simulink model "SatelliteDynamicsAndKinematics_Model"  (R2024a)
settings: Solver=VariableStepAuto  StartTime=0.0  StopTime=10.0  RelTol=1e-3
values from neighbouring files (symbols this model uses):
  sat = satellite_params()    [init_SAR_AOCS.m]
undefined symbols (not defined in the file or in its folder): initial
libraries: sharedtransform x3, matrix_library x1, aerolibutil x1, simulink_extras x1
settings Model: Creator=hendr  LastModifiedBy=hendr

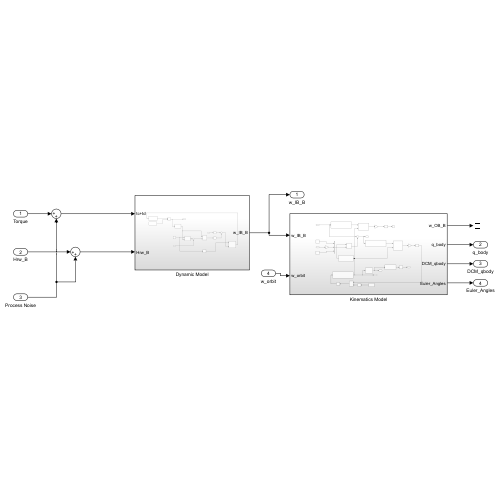
[thumbnail: Simulink's stored preview of the top-level diagram]
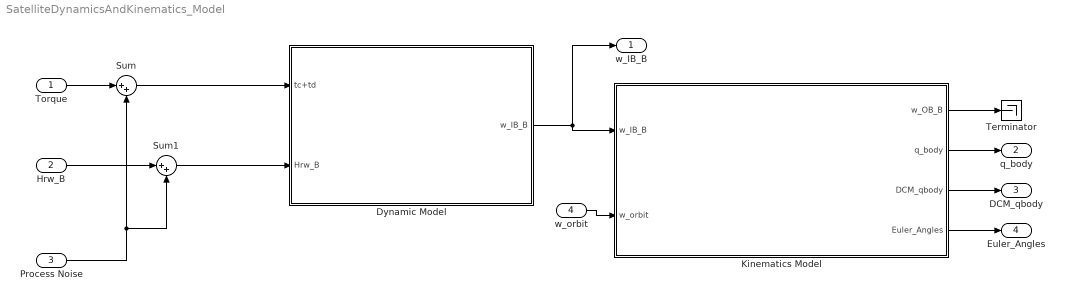
== system SatelliteDynamicsAndKinematics_Model ==
  Torque : Inport
  Hrw_B : Inport  Port=2
  Process Noise : Inport  Port=3
  w_orbit : Inport  Port=4
  Dynamic Model : Subsystem
  Kinematics Model : Subsystem
  Sum : Sum  Inputs=|++
  Sum1 : Sum  Inputs=|++
  Terminator : Terminator
  w_IB_B : Outport
  q_body : Outport  Port=2
  DCM_qbody : Outport  Port=3
  Euler_Angles : Outport  Port=4
  wires:
  Torque/1 -> Sum/1
  Process Noise/1 -> Sum1/2, Sum/2
  Hrw_B/1 -> Sum1/1
  Sum/1 -> Dynamic Model/1(tc+td)
  Sum1/1 -> Dynamic Model/2(Hrw_B)
  Dynamic Model/1(w_IB_B) -> w_IB_B/1, Kinematics Model/1(w_IB_B)
  w_orbit/1 -> Kinematics Model/2(w_orbit)
  Kinematics Model/2(q_body) -> q_body/1
  Kinematics Model/1(w_OB_B) -> Terminator/1
  Kinematics Model/3(DCM_qbody) -> DCM_qbody/1
  Kinematics Model/4(Euler_Angles) -> Euler_Angles/1

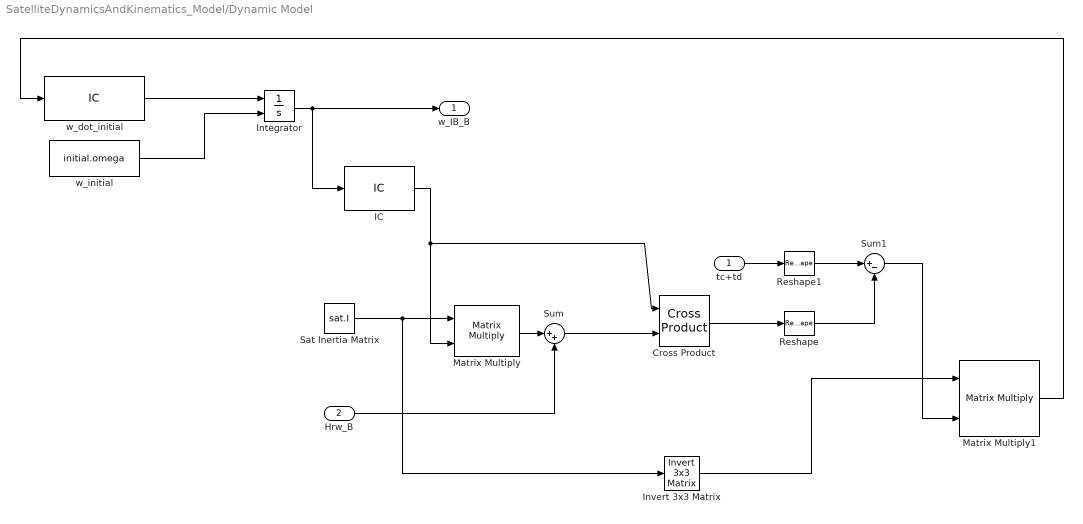
== system SatelliteDynamicsAndKinematics_Model/Dynamic Model ==
  tc+td : Inport
  Hrw_B : Inport  Port=2
  Cross Product : matrix_library/Cross Product
  IC : InitialCondition  Value=initial.omega
  Integrator : Integrator  InitialConditionSource=external
  Invert 3x3 Matrix : aerolibutil/Invert  3x3 Matrix
  Matrix Multiply : Product  Multiplication=Matrix(*)
  Matrix Multiply1 : Product  Multiplication=Matrix(*)
  Reshape : Reshape  OutputDimensionality=Column vector (2-D)
  Reshape1 : Reshape  OutputDimensionality=Column vector (2-D)
  Sat Inertia Matrix : Constant  Value=sat.I
  Sum : Sum  Inputs=|++
  Sum1 : Sum  Inputs=|+-
  w_dot_initial : InitialCondition  Value=initial.omegadot
  w_initial : Constant  Value=initial.omega
  w_IB_B : Outport
  wires:
  Sat Inertia Matrix/1 -> Invert 3x3 Matrix/1, Matrix Multiply/1
  Matrix Multiply/1 -> Sum/1
  Hrw_B/1 -> Sum/2
  Sum/1 -> Cross Product/2
  w_initial/1 -> Integrator/2
  w_dot_initial/1 -> Integrator/1
  Integrator/1 -> IC/1, w_IB_B/1
  IC/1 -> Cross Product/1, Matrix Multiply/2
  Cross Product/1 -> Reshape/1
  Reshape/1 -> Sum1/2
  Sum1/1 -> Matrix Multiply1/2
  Invert 3x3 Matrix/1 -> Matrix Multiply1/1
  tc+td/1 -> Reshape1/1
  Reshape1/1 -> Sum1/1
  Matrix Multiply1/1 -> w_dot_initial/1

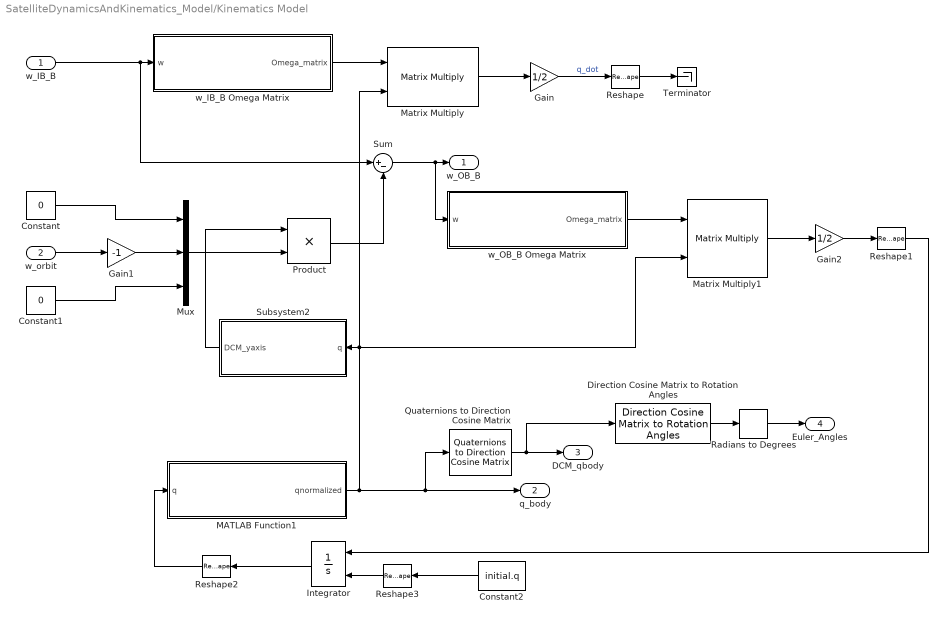
== system SatelliteDynamicsAndKinematics_Model/Kinematics Model ==
  w_IB_B : Inport
  w_orbit : Inport  Port=2
  Constant : Constant  Value=0
  Constant1 : Constant  Value=0
  Constant2 : Constant  Value=initial.q
  Direction Cosine Matrix to Rotation Angles : sharedtransform/Direction Cosine Matrix to Rotation Angles  rotationOrder=ZYX  aMode=aMode  action=None  tolerance=eps(2)
      settings: LibrarySourceBlock=|
      | aerolibtransform2/Direction Cosine Matrix
      | to Rotation Angles
  Gain : Gain  Gain=1/2
  Gain1 : Gain  Gain=-1
  Gain2 : Gain  Gain=1/2
  Integrator : Integrator  InitialConditionSource=external
  MATLAB Function1 : MATLAB Function  TreatAsAtomicUnit=on
  Matrix Multiply : Product  Multiplication=Matrix(*)
  Matrix Multiply1 : Product  Multiplication=Matrix(*)
  Mux : Mux  Inputs=3
  Product : Product
  Quaternions to Direction Cosine Matrix : sharedtransform/Quaternions to  Direction Cosine Matrix  aMode=aMode
      settings: LibrarySourceBlock=|
      | aerolibtransform2/Quaternions to
      | Direction Cosine Matrix
  Radians to Degrees : simulink_extras/Transformations/Radians to Degrees
  Reshape{,1..3} (4 alike) : Reshape  OutputDimensionality=Column vector (2-D)
  Subsystem2 : Subsystem
  Sum : Sum  Inputs=|+-
  Terminator : Terminator
  w_IB_B Omega Matrix : MATLAB Function  TreatAsAtomicUnit=on
  w_OB_B Omega Matrix : MATLAB Function  TreatAsAtomicUnit=on
  w_OB_B : Outport
  q_body : Outport  Port=2
  DCM_qbody : Outport  Port=3
  Euler_Angles : Outport  Port=4
  wires:
  w_IB_B/1 -> Sum/1, w_IB_B Omega Matrix/1(w)
  w_IB_B Omega Matrix/1(Omega_matrix) -> Matrix Multiply/1
  Matrix Multiply/1 -> Gain/1
  Gain/1 -> Reshape/1  "q_dot"
  Reshape/1 -> Terminator/1
  w_orbit/1 -> Gain1/1
  Constant/1 -> Mux/1
  Constant1/1 -> Mux/3
  Gain1/1 -> Mux/2
  Mux/1 -> Product/2
  Product/1 -> Sum/2
  Sum/1 -> w_OB_B Omega Matrix/1(w), w_OB_B/1
  w_OB_B Omega Matrix/1(Omega_matrix) -> Matrix Multiply1/1
  MATLAB Function1/1(qnormalized) -> Quaternions to Direction Cosine Matrix/1, q_body/1, Matrix Multiply1/2, Matrix Multiply/2, Subsystem2/1(q)
  Subsystem2/1(DCM_yaxis) -> Product/1
  Matrix Multiply1/1 -> Gain2/1
  Reshape1/1 -> Integrator/1
  Gain2/1 -> Reshape1/1
  Reshape3/1 -> Integrator/2
  Integrator/1 -> Reshape2/1
  Reshape2/1 -> MATLAB Function1/1(q)
  Constant2/1 -> Reshape3/1
  Quaternions to Direction Cosine Matrix/1 -> Direction Cosine Matrix to Rotation Angles/1, DCM_qbody/1
  Direction Cosine Matrix to Rotation Angles/1 -> Radians to Degrees/1
  Radians to Degrees/1 -> Euler_Angles/1

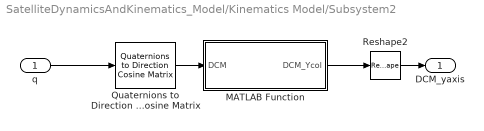
== system SatelliteDynamicsAndKinematics_Model/Kinematics Model/Subsystem2 ==
  q : Inport
  MATLAB Function : MATLAB Function  TreatAsAtomicUnit=on
  Quaternions to Direction Cosine Matrix : sharedtransform/Quaternions to  Direction Cosine Matrix  aMode=aMode
  Reshape2 : Reshape  OutputDimensionality=Column vector (2-D)
  DCM_yaxis : Outport  VectorParamsAs1DForOutWhenUnconnected=off
  wires:
  q/1 -> Quaternions to Direction Cosine Matrix/1
  Quaternions to Direction Cosine Matrix/1 -> MATLAB Function/1(DCM)
  MATLAB Function/1(DCM_Ycol) -> Reshape2/1
  Reshape2/1 -> DCM_yaxis/1

== matlab function SatelliteDynamicsAndKinematics_Model/Kinematics Model/w_IB_B Omega Matrix ==
  data: w input; Omega_matrix output
function Omega_matrix = quat_omega_matrix(w)

wx = w(1);
wy = w(2);
wz = w(3);

y = [ 0,  -wx, -wy, -wz;
      wx,   0,  wz, -wy;
      wy, -wz,   0,  wx;
      wz,  wy, -wx,   0];
end

== matlab function SatelliteDynamicsAndKinematics_Model/Kinematics Model/w_OB_B Omega Matrix ==
  data: w input; Omega_matrix output
function Omega_matrix = quat_omega_matrix(w)

wx = w(1);
wy = w(2);
wz = w(3);

y = [ 0,  -wx, -wy, -wz;
      wx,   0,  wz, -wy;
      wy, -wz,   0,  wx;
      wz,  wy, -wx,   0];
end

== matlab function SatelliteDynamicsAndKinematics_Model/Kinematics Model/Subsystem2/MATLAB Function ==
  data: DCM input; DCM_Ycol output
function DCM_Ycol = fcn(DCM)
DCM_2 = DCM(:,2); % orbit frame Y axis
end

== matlab function SatelliteDynamicsAndKinematics_Model/Kinematics Model/MATLAB Function1 ==
  data: q input; qnormalized output
function qnormalized = qnorm(q)

qnorm = norm(q);

if qnorm < 1e-12 % Protects from divide by 0 errors
    qnormalized = [1; 0; 0; 0]; % identity quaternion
else
    qnormalized = q / qnorm;
end

end
